simulink model "Simulation_WTA"  (R2020a)
settings: Solver=ode45  StartTime=0.0  StopTime=100  RelTol=1e-3  EnableMultiTasking=on
undefined symbols (not defined in the file): n
(part 5 of 5)

== matlab function Simulation_WTA/MATLAB Function3 ==
  data: x output; x input; v_dot output
function [x,v_dot]= fcn(x)
n=7;
for i=1:1:n*n
   if x(i)>=0.5
       x(i) = 1;
   else
       x(i) = 0;
   end
end
v_dot = (-1)*ones(2*n,1);
for i=1:1:n
    for j=1:1:n
        v_dot(i) = v_dot(i)+x(n*(i-1)+j);
        v_dot(n+i) = v_dot(n+i)+x(n*(j-1)+i);
    end
end
